simulink model "Mdl4ws_TS9"  (Simulink 8.5)
settings: Solver=ode45  SolverMode=SingleTasking  StartTime=0  StopTime=12  FixedStep=0.002  RelTol=1e-3  AbsTol=1e-6
libraries: Solver_SF x1
settings Model: Creator=bduprey  LastModifiedBy=mkhan  CovHtmlReporting=off  CovSFcnEnable=off  ExtModeTrigMode=oneshot  ExtModeArmWhenConnect=off
settings DataIOCC: LimitDataPoints=off
settings OptimizationCC: BlockReduction=off  BooleanDataType=off
settings DebuggingCC: SaveWithParameterizedLinksMsg=none  SignalResolutionControl=TryResolveAllWithWarning  MultiTaskDSMMsg=warning  MultiTaskCondExecSysMsg=none  FcnCallInpInsideContextMsg=EnableAllAsWarning
settings HardwareCC: TargetUnknown=on
settings RTWCC: TemplateMakefile=grt_vc.tmf
settings GRTTargetCC: TargetFcnLib=ansi_tfl_tmw.mat

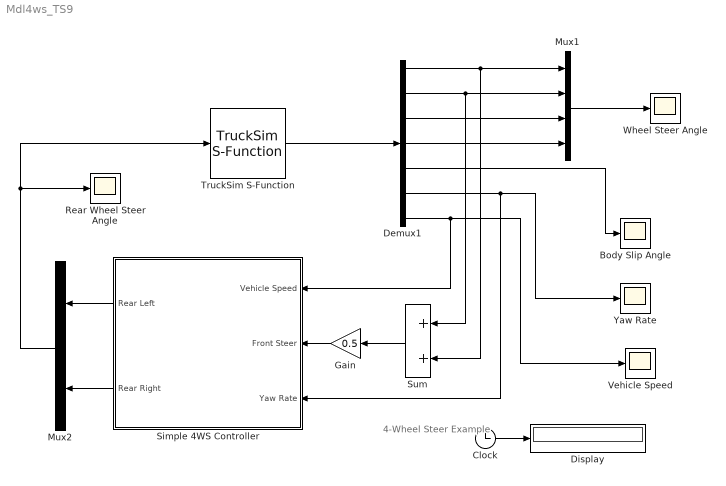
== system Mdl4ws_TS9 ==
  note: 4-Wheel Steer Example
  Body Slip Angle : Scope
      settings: TimeRange=auto  TickLabels=on  MaxDataPoints=5000  SaveToWorkspace=off  SaveName=ScopeData  YMin=-1  YMax=1.5  SampleTime=-1  DataFormat=Array  Decimation=10
  Clock : Clock
  Demux1 : Demux  Outputs=[1 1 1 1 1 1 1]
      settings: DisplayOption=none
  Display : Display
      settings: Format=bank  Decimation=100
  Gain : Gain  Gain=0.5  SaturateOnIntegerOverflow=on  OutDataTypeStr=Inherit: Same as input  ParamDataTypeStr=Inherit: Same as input
  Mux1 : Mux
  Mux2 : Mux  Inputs=2
  Rear Wheel Steer Angle : Scope
      settings: TimeRange=auto  TickLabels=on  MaxDataPoints=5000  SaveToWorkspace=off  SaveName=ScopeData  YMin=-2  YMax=2  SampleTime=-1  DataFormat=Array  Decimation=10
  Simple 4WS Controller : Subsystem  mask{m=7960, lf=3.102, lr=1.388, Cf=162521, Cr=139081}
      mask prompts: m "body mass (kg)"; lf "length f-G (m)"; lr "length r-G (m)"; Cf "conering power f  (N/rad)"; Cr "conering power r  (N/rad)"
  Sum : Sum  InputSameDT=on  SaturateOnIntegerOverflow=on  OutDataTypeStr=Inherit: Same as first input
  TruckSim S-Function : Solver_SF/TruckSim S-Function  Priority=1  SIMFILE=simfile.sim  Run_RTs=off  vs_state_ind=Run  StopMode_ind=Vehicle Model
  Vehicle Speed : Scope
      settings: TimeRange=12  TickLabels=on  MaxDataPoints=5000  SaveToWorkspace=off  SaveName=ScopeData  YMin=99.5  YMax=100.5  SampleTime=-1  DataFormat=Array  Decimation=10
  Wheel Steer Angle : Scope
      settings: TimeRange=auto  TickLabels=on  MaxDataPoints=5000  SaveToWorkspace=off  SaveName=ScopeData  YMin=-10  YMax=10  SampleTime=-1  DataFormat=Array  Decimation=10
  Yaw Rate : Scope
      settings: TimeRange=auto  TickLabels=on  MaxDataPoints=5000  SaveToWorkspace=off  SaveName=ScopeData  YMin=-10  YMax=10  SampleTime=-1  DataFormat=Array  Decimation=10
  wires:
  Sum/1 -> Gain/1
  Gain/1 -> Simple 4WS Controller/2(Front Steer)
  Mux1/1 -> Wheel Steer Angle/1
  Demux1/1 -> Sum/2, Mux1/1
  Demux1/2 -> Sum/1, Mux1/2
  Demux1/3 -> Mux1/3
  Demux1/4 -> Mux1/4
  Demux1/5 -> Body Slip Angle/1
  Demux1/6 -> Simple 4WS Controller/3(Yaw Rate), Yaw Rate/1
  Demux1/7 -> Simple 4WS Controller/1(Vehicle Speed), Vehicle Speed/1
  TruckSim S-Function/1 -> Demux1/1
  Simple 4WS Controller/1(Rear Left) -> Mux2/1
  Simple 4WS Controller/2(Rear Right) -> Mux2/2
  Clock/1 -> Display/1
  Mux2/1 -> Rear Wheel Steer Angle/1, TruckSim S-Function/1

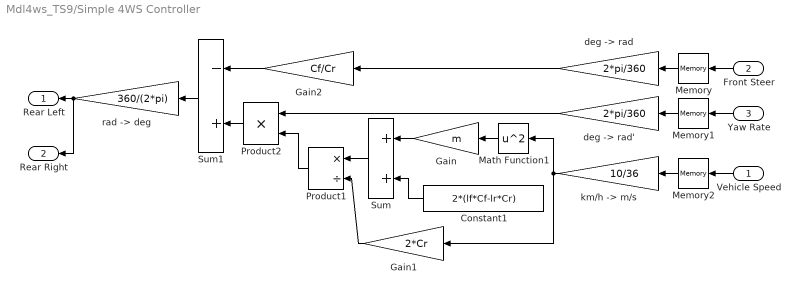
== system Mdl4ws_TS9/Simple 4WS Controller ==
  Vehicle Speed : Inport
  Front Steer : Inport  Port=2
  Yaw Rate : Inport  Port=3
  Constant1 : Constant  Value=2*(lf*Cf-lr*Cr)
  Gain : Gain  Gain=m  SaturateOnIntegerOverflow=on  OutDataTypeStr=Inherit: Same as input  ParamDataTypeStr=Inherit: Same as input
  Gain1 : Gain  Gain=2*Cr  SaturateOnIntegerOverflow=on  OutDataTypeStr=Inherit: Same as input  ParamDataTypeStr=Inherit: Same as input
  Gain2 : Gain  Gain=Cf/Cr  SaturateOnIntegerOverflow=on  OutDataTypeStr=Inherit: Same as input  ParamDataTypeStr=Inherit: Same as input
  Math Function1 : Math  Operator=square  SaturateOnIntegerOverflow=on
  Memory : Memory
  Memory1 : Memory
  Memory2 : Memory  X0=80
  Product1 : Product  Inputs=*/  InputSameDT=on  RndMeth=Zero  SaturateOnIntegerOverflow=on  OutDataTypeStr=Inherit: Same as first input
  Product2 : Product  InputSameDT=on  RndMeth=Zero  SaturateOnIntegerOverflow=on  OutDataTypeStr=Inherit: Same as first input
  Sum : Sum  InputSameDT=on  SaturateOnIntegerOverflow=on  OutDataTypeStr=Inherit: Same as first input
  Sum1 : Sum  Inputs=-+  InputSameDT=on  SaturateOnIntegerOverflow=on  OutDataTypeStr=Inherit: Same as first input
  "deg -> rad" : Gain  Gain=2*pi/360  SaturateOnIntegerOverflow=on  OutDataTypeStr=Inherit: Same as input  ParamDataTypeStr=Inherit: Same as input
  "deg -> rad'" : Gain  Gain=2*pi/360  SaturateOnIntegerOverflow=on  OutDataTypeStr=Inherit: Same as input  ParamDataTypeStr=Inherit: Same as input
  "km/h -> m/s" : Gain  Gain=10/36  SaturateOnIntegerOverflow=on  OutDataTypeStr=Inherit: Same as input  ParamDataTypeStr=Inherit: Same as input
  "rad -> deg" : Gain  Gain=360/(2*pi)  SaturateOnIntegerOverflow=on  OutDataTypeStr=Inherit: Same as input  ParamDataTypeStr=Inherit: Same as input
  Rear Left : Outport  InitialOutput=0
  Rear Right : Outport  Port=2  InitialOutput=0
  wires:
  Product1/1 -> Product2/2
  Product2/1 -> Sum1/2
  Gain1/1 -> Product1/2
  Constant1/1 -> Sum/2
  Math Function1/1 -> Gain/1
  Gain/1 -> Sum/1
  Sum/1 -> Product1/1
  Gain2/1 -> Sum1/1
  "km/h -> m/s"/1 -> Math Function1/1, Gain1/1
  "deg -> rad'"/1 -> Product2/1
  "deg -> rad"/1 -> Gain2/1
  Sum1/1 -> "rad -> deg"/1
  Front Steer/1 -> Memory/1
  Memory/1 -> "deg -> rad"/1
  Yaw Rate/1 -> Memory1/1
  Memory1/1 -> "deg -> rad'"/1
  Vehicle Speed/1 -> Memory2/1
  Memory2/1 -> "km/h -> m/s"/1
  "rad -> deg"/1 -> Rear Left/1, Rear Right/1
